simulink model "ss_state_feedback_control"  (R2022a)
settings: Solver=VariableStepAuto  StartTime=0.0  StopTime=10.0  MaxStep=1e-3  RelTol=1e-3
values from neighbouring files (symbols this model uses):
  A0 = [-1 1;0 0]    [delayDependent_Lyapunov_Krasovskii_analysis.m]    (also in delayDependent_Razumikhin_analysis.m)
  B = [0;1]    [delayDependent_Lyapunov_Krasovskii_analysis.m]    (also in delayDependent_Razumikhin_analysis.m)
  C = [1 0]    [delayDependent_Lyapunov_Krasovskii_analysis.m]    (also in delayDependent_Razumikhin_analysis.m)
  K = -acker(A0,B,[-3 -2])    [delayDependent_Lyapunov_Krasovskii_analysis.m]    (also in delayDependent_Razumikhin_analysis.m = acker(A0,B,[-3 -2]))
settings Model: Creator=aaron  LastModifiedBy=aaron

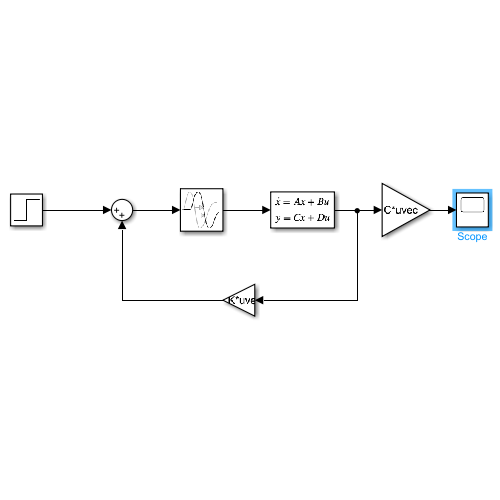
[thumbnail: Simulink's stored preview of the top-level diagram]
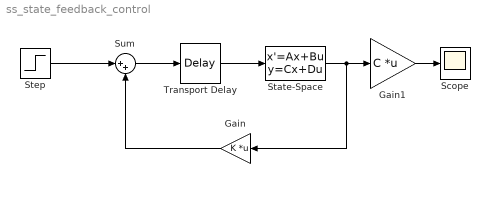
== system ss_state_feedback_control ==
  Gain : Gain  Gain=K  Multiplication=Matrix(K*u) (u vector)
  Gain1 : Gain  Gain=C  Multiplication=Matrix(K*u) (u vector)
  Scope : Scope
  State-Space : StateSpace  A=A0  B=B  C=eye(2)  D=zeros(2,1)  InitialCondition=0
  Step : Step  Time=0  SampleTime=0
  Sum : Sum  Inputs=|++
  Transport Delay : TransportDelay  DelayTime=0.353
  wires:
  Step/1 -> Sum/1
  Sum/1 -> Transport Delay/1
  Gain1/1 -> Scope/1
  Transport Delay/1 -> State-Space/1
  State-Space/1 -> Gain/1, Gain1/1
  Gain/1 -> Sum/2
